simulink model "boat_simulator_ros_node"  (R2020a)
settings: Solver=FixedStepAuto  StartTime=0.0  StopTime=inf  RelTol=1e-3
PreLoadFcn:
  | % ROS setup
  | rosshutdown;
  | ipAddr = '';
  | rosinit(ipAddr)
  | 
  | % Sample times
  | sampleTime = 0.2;
  | 
  | % Control parameters
  | ctrlParam1 = 2;
  | ctrlParam2 = 3.5;
undefined symbols (not defined in the file or in its folder): GpsAisGroundspeedKnots, GpsCanGroundspeedKnots, GpsCanLatitudeDegrees, GpsCanLongitudeDegrees, GpsCanTrueHeadingDegrees, par, WindSensor1AngleDegrees, WindSensor1SpeedKnots, WindSensor2AngleDegrees, WindSensor2SpeedKnots, WindSensor3AngleDegrees, WindSensor3SpeedKnots
libraries: simulink_extras x5, robotlib x4, UBCSailbotBlocks x1
settings Model: Creator=scastro  LastModifiedBy=bruce
settings DataIOCC: ReturnWorkspaceOutputs=off
settings OptimizationCC: PassReuseOutputArgsAs=Individual arguments  MaxStackSize=64  EfficientTunableParamExpr=on
settings DebuggingCC: ParameterTunabilityLossMsg=error  ArithmeticOperatorsInVariantConditions=warning
settings HardwareCC: ProdBitPerLong=64  ProdHWDeviceType=Intel->x86-64 (Linux 64)
settings SFSimCC: SimUseLocalCustomCode=off  MATLABDynamicMemAlloc=off  CustomCodeUndefinedFunction=UseInterfaceOnly
settings RTWCC: SystemTargetFile=ert.tlc  HardwareBoard=Robot Operating System (ROS)  TemplateMakefile=ert_default_tmf  GenerateReport=on  RTWUseLocalCustomCode=off  Toolchain=Catkin  IncludeHyperlinkInReport=on  LaunchReport=on  PortableWordSizes=on  TargetLang=C++  GenerateTraceInfo=on  GenerateTraceReport=on  GenerateTraceReportSl=on  GenerateTraceReportSf=on  GenerateTraceReportEml=on
settings CodeAppCC: ForceParamTrailComments=on  IgnoreCustomStorageClasses=off  OperatorAnnotations=on  SimulinkDataObjDesc=on  SFDataObjDesc=on  InsertBlockDesc=on
settings TargetCC: MultiwordLength=256  ParMdlRefBuildCompliant=on  ConcurrentExecutionCompliant=on  CombineOutputUpdateFcns=on  ERTCustomFileBanners=on  RemoveResetFunc=on  SupportVariableSizeSignals=on  MATLABClassNameForMDSCustomization=Simulink.SoftwareTarget.ERTCustomization  ModelStepFunctionPrototypeControlCompliant=on  CPPClassGenCompliant=on  GRTInterface=off  UseToolchainInfoCompliant=on

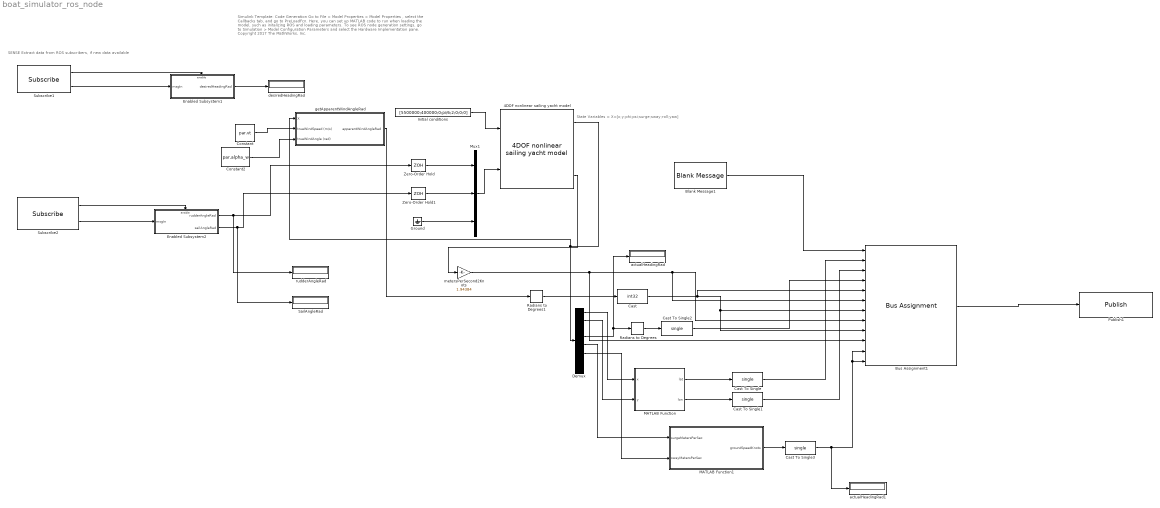
== system boat_simulator_ros_node ==
  note: State Variables = X=[x;y;phi;psi;surge;sway;roll;yaw]
  note: SENSE
      | Extract data from ROS subscribers, if new data available
  note: Simulink Template: Code Generation
      |
      | Go to File > Model Properties > Model Properties , select the Callbacks tab, and go to PreLoadFcn. Here, you can set up MATLAB code to run when loading the model, such as initalizing ROS and loading parameters.
      |
      | To see ROS node generation settings, go to Simulation > Model Configuration Parameters and select the Hardware Implementation pane.
      |
      | Copyright 2017 The MathWorks, Inc.
  4DOF nonlinear sailing yacht model : UBCSailbotBlocks/4DOF nonlinear sailing yacht model  SystemSampleTime=-1  Latency=0  AutoFrameSizeCalculation=off
  Blank Message1 : robotlib/Blank Message  messageClass=Message  entityType=sailbot_msg/Sensors  messageType=sailbot_msg/Sensors  SampleTime=inf
  Bus Assignment1 : BusAssignment  AssignedSignals=GpsCanLatitudeDegrees,GpsCanLongitudeDegrees,GpsCanTrueHeadingDegrees,WindSensor3AngleDegrees,WindSensor3SpeedKnots,WindSensor2AngleDegrees,WindSensor2SpeedKnots,WindSensor1AngleDegrees,WindSensor1SpeedKnots,GpsCanGroundspeedKnots,GpsAisGroundspeedKnots
  Cast : DataTypeConversion  OutDataTypeStr=int32
  Cast To Single{,1..3} (4 alike) : DataTypeConversion  OutDataTypeStr=single
  Constant : Constant  Value=par.vt
  Constant2 : Constant  Value=par.alpha_w  VectorParams1D=off
  Demux : Demux  Outputs=8
  Enabled Subsystem1 : Subsystem  TreatAsAtomicUnit=on
  Enabled Subsystem2 : Subsystem  TreatAsAtomicUnit=on
  Ground : Ground
  Initial conditions : Constant  Value=[5500000;400000;0;pi/6;2;0;0;0]
  MATLAB Function : MATLAB Function  TreatAsAtomicUnit=on
  MATLAB Function1 : MATLAB Function  TreatAsAtomicUnit=on
  Mux1 : Mux  Inputs=3
  Publish1 : robotlib/Publish  topicSource=Specify your own  topic=/sensors  messageType=sailbot_msg/Sensors  messageQueueLength=1
  Radians to Degrees : simulink_extras/Transformations/Radians to Degrees
  Radians to Degrees1 : simulink_extras/Transformations/Radians to Degrees
  SailAngleRad : Display
  Subscribe1 : robotlib/Subscribe  topicSource=Specify your own  topic=/desired_heading_degrees  messageType=sailbot_msg/heading  sampleTime=-1  messageQueueLength=1
  Subscribe2 : robotlib/Subscribe  topicSource=Specify your own  topic=/rudder_winch_actuation_angle  messageType=sailbot_msg/actuation_angle  sampleTime=-1  messageQueueLength=1
  Zero-Order Hold : ZeroOrderHold  SampleTime=0.1
  Zero-Order Hold1 : ZeroOrderHold  SampleTime=0.1
  actualHeadingRad : Display
  actualHeadingRad1 : Display
  desiredHeadingRad : Display
  getApparentWindAngleRad : Subsystem  AncestorBlock=UBCSailbotBlocks/controller using true wind speed and angle
  metersPerSecond2Knots : Gain  Gain=1.94384  OutDataTypeStr=single
  rudderAngleRad : Display
  wires:
  Subscribe1/2 -> Enabled Subsystem1/1(msgIn)
  Subscribe1/1 -> Enabled Subsystem1/Enable
  Bus Assignment1/1 -> Publish1/1
  4DOF nonlinear sailing yacht model/1 -> Demux/1, getApparentWindAngleRad/1(X)
  Initial conditions/1 -> 4DOF nonlinear sailing yacht model/1
  Blank Message1/1 -> Bus Assignment1/1
  Mux1/1 -> 4DOF nonlinear sailing yacht model/2
  Constant2/1 -> getApparentWindAngleRad/3(trueWindAngle (rad))
  Demux/1 -> MATLAB Function/1(x)
  Demux/2 -> MATLAB Function/2(y)
  Zero-Order Hold/1 -> Mux1/1
  Zero-Order Hold1/1 -> Mux1/2
  Ground/1 -> Mux1/3
  Constant/1 -> getApparentWindAngleRad/2(trueWindSpeed (m/s))
  Demux/4 -> Radians to Degrees/1, actualHeadingRad/1
  Enabled Subsystem1/1(desiredHeadingRad) -> desiredHeadingRad/1
  Radians to Degrees1/1 -> Cast/1
  4DOF nonlinear sailing yacht model/3 -> metersPerSecond2Knots/1
  MATLAB Function/1(lat) -> Cast To Single/1
  MATLAB Function/2(lon) -> Cast To Single1/1
  Radians to Degrees/1 -> Cast To Single2/1
  Cast/1 -> Bus Assignment1/9, Bus Assignment1/7, Bus Assignment1/5
  metersPerSecond2Knots/1 -> Bus Assignment1/6, Bus Assignment1/8, Bus Assignment1/10
  Cast To Single/1 -> Bus Assignment1/2
  Cast To Single1/1 -> Bus Assignment1/3
  Cast To Single2/1 -> Bus Assignment1/4
  Demux/5 -> MATLAB Function1/1(surgeMetersPerSec)
  Demux/6 -> MATLAB Function1/2(swayMetersPerSec)
  getApparentWindAngleRad/1(apparentWindAngleRad) -> Radians to Degrees1/1
  Subscribe2/1 -> Enabled Subsystem2/Enable
  Subscribe2/2 -> Enabled Subsystem2/1(msgIn)
  Enabled Subsystem2/1(rudderAngleRad) -> rudderAngleRad/1, Zero-Order Hold/1
  Enabled Subsystem2/2(sailAngleRad) -> SailAngleRad/1, Zero-Order Hold1/1
  MATLAB Function1/1(groundSpeedKnots) -> Cast To Single3/1
  Cast To Single3/1 -> actualHeadingRad1/1, Bus Assignment1/12, Bus Assignment1/11

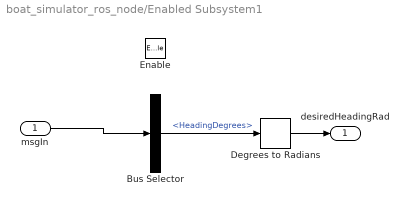
== system boat_simulator_ros_node/Enabled Subsystem1 ==
  msgIn : Inport
  Enable : EnablePort
  Bus Selector : BusSelector  OutputSignals=HeadingDegrees
  Degrees to Radians : simulink_extras/Transformations/Degrees to Radians
  desiredHeadingRad : Outport  VectorParamsAs1DForOutWhenUnconnected=off
  wires:
  msgIn/1 -> Bus Selector/1
  Bus Selector/1 -> Degrees to Radians/1  "<HeadingDegrees>"
  Degrees to Radians/1 -> desiredHeadingRad/1

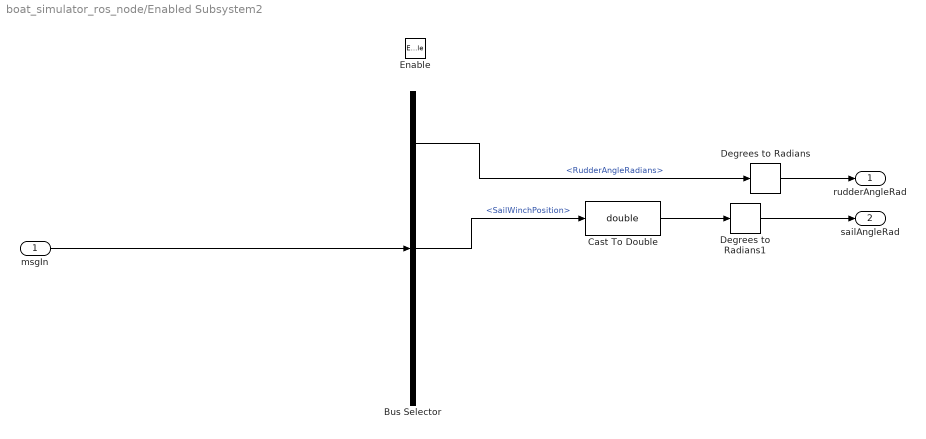
== system boat_simulator_ros_node/Enabled Subsystem2 ==
  msgIn : Inport
  Enable : EnablePort
  Bus Selector : BusSelector  OutputSignals=RudderAngleRadians,SailWinchPosition,JibWinchPosition
  Cast To Double : DataTypeConversion  OutDataTypeStr=double
  Degrees to Radians : simulink_extras/Transformations/Degrees to Radians
  Degrees to Radians1 : simulink_extras/Transformations/Degrees to Radians
  rudderAngleRad : Outport  VectorParamsAs1DForOutWhenUnconnected=off
  sailAngleRad : Outport  Port=2  VectorParamsAs1DForOutWhenUnconnected=off
  wires:
  msgIn/1 -> Bus Selector/1
  Bus Selector/1 -> Degrees to Radians/1  "<RudderAngleRadians>"
  Degrees to Radians/1 -> rudderAngleRad/1
  Bus Selector/2 -> Cast To Double/1  "<SailWinchPosition>"
  Degrees to Radians1/1 -> sailAngleRad/1
  Cast To Double/1 -> Degrees to Radians1/1

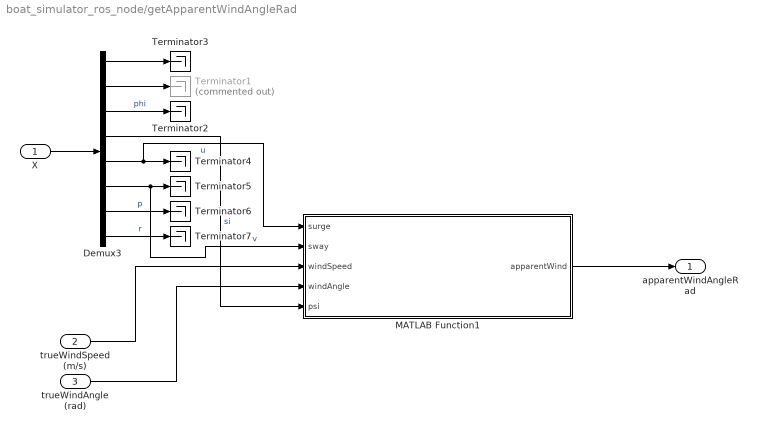
== system boat_simulator_ros_node/getApparentWindAngleRad ==
  X : Inport
  trueWindSpeed (m/s) : Inport  Port=2
  trueWindAngle (rad) : Inport  Port=3
  Demux3 : Demux  Outputs=8
  MATLAB Function1 : MATLAB Function  TreatAsAtomicUnit=on
  Terminator1 : Terminator  Commented=on
  Terminator{2..7} (6 alike) : Terminator
  apparentWindAngleRad : Outport
  wires:
  MATLAB Function1/1(apparentWind) -> apparentWindAngleRad/1
  trueWindAngle (rad)/1 -> MATLAB Function1/4(windAngle)
  trueWindSpeed (m/s)/1 -> MATLAB Function1/3(windSpeed)
  Demux3/8 -> Terminator7/1  "r"
  Demux3/7 -> Terminator6/1  "p"
  Demux3/6 -> Terminator5/1, MATLAB Function1/2(sway)  "v"
  Demux3/5 -> Terminator4/1, MATLAB Function1/1(surge)  "u"
  Demux3/3 -> Terminator2/1  "phi"
  Demux3/2 -> Terminator1/1
  Demux3/1 -> Terminator3/1
  X/1 -> Demux3/1
  Demux3/4 -> MATLAB Function1/5(psi)  "si"

== matlab function boat_simulator_ros_node/MATLAB Function1 ==
  data: surgeMetersPerSec input; groundSpeedKnots output; swayMetersPerSec input
function groundSpeedKnots = getGroundSpeedKnots(surgeMetersPerSec, swayMetersPerSec)

KNOTS_PER_METERS_PER_SECOND = 1.94384;

groundSpeedKnots = sqrt(surgeMetersPerSec^2 + swayMetersPerSec^2)* KNOTS_PER_METERS_PER_SECOND;

== matlab function boat_simulator_ros_node/MATLAB Function ==
  data: x input; lat output; y input; lon output
function [lat, lon] = metersToLatLonWrapper(x, y)
coder.extrinsic('metersToLatLon'); 
lat = NaN;
lon = NaN;
[lat,lon] = metersToLatLon(x,y);

== matlab function boat_simulator_ros_node/getApparentWindAngleRad/MATLAB Function1 ==
  data: surge input; apparentWind output; sway input; windSpeed input; windAngle input; psi input
function apparentWind = getApparentWindAngleWrapper(surge, sway, windSpeed, windAngle, psi)

apparentWind = getApparentWindAngle(surge, sway, windSpeed, windAngle, psi);
